simulink model "batt_test"  (Simulink 7.8)
settings: Solver=ode3  StartTime=0.0  StopTime=20  FixedStep=80e-6  RelTol=1e-3
PostLoadFcn:
  | Ts=80e-6;
InitFcn:
  | Ts=80e-6;
values from neighbouring files (symbols this model uses):
  batt_esr = (max_power*0.01)/(max_power/Vdc_nom)^2    [BES_init.m]
  C = IacRMS*18e-6    [BES_init.m]
  f = 60    [global_parameters.m]
  I_ki = 0.03    [BES_init.m]
  I_kp = 0.05    [BES_init.m]
  Iac_max = IGBT_currents(possible_currents(1))    [BES_init.m]
  Id_at_max = 3*max_pow*(2/3)/Vd_at_max    [BES_init.m]
  Iq_at_max = 3*max_pow*(2/3)/Vq_at_max    [BES_init.m]
  L = Vdc_nom/(IacRMS*0.2/(2/fs))    [BES_init.m]
  PLL_Ki = 0.001*30    (= 0.03)    [BES_init.m]
  PLL_Kp = .001*30    (= 0.03)    [BES_init.m]
  PLL_time_step = Ts    (= 8e-05)    [global_parameters.m]
  Roff = 1e7    (= 10000000)    [BES_init.m]
  Td_es_min = Ts    (= 8e-05)    [global_parameters.m]
  Tds = Ts    (= 8e-05)    [global_parameters.m]
  Vdc_max = IGBT_voltages(possible_voltages(1))    [BES_init.m]
undefined symbols (not defined in the file or in its folder): D, DiscIntNeverNeededParam
libraries: simulink x25, powerlib x20, simulink_extras x10, cstextras x9, powerlib_extras x8, modbus_lib x6, dynamic_load_lib x1, dspsigops x1
(part 2 of 2)

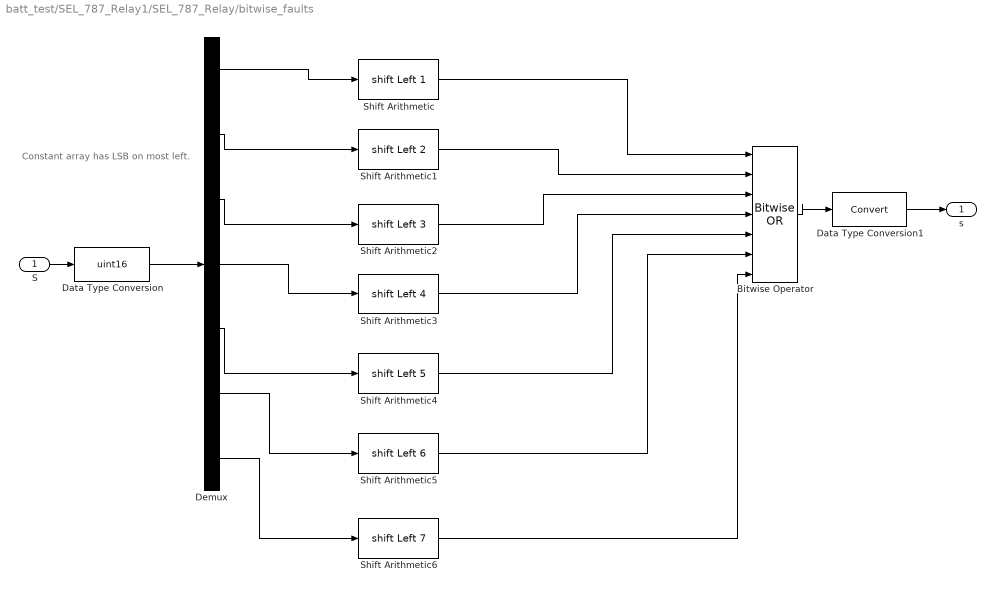
== system batt_test/SEL_787_Relay1/SEL_787_Relay/bitwise_faults ==
  note: Constant array has LSB on most left.
  S : Inport
  Bitwise Operator : simulink/Logic and Bit Operations/Bitwise Operator  logicop=OR  UseBitMask=off  NumInputPorts=7  BitMask=bin2dec('11011001')  BitMaskRealWorld=Stored Integer
  Data Type Conversion : DataTypeConversion  OutDataTypeStr=uint16
  Data Type Conversion1 : DataTypeConversion
  Demux : Demux  Outputs=7
  Shift Arithmetic : ArithShift  BitShiftNumber=1  BitShiftDirection=Left
  Shift Arithmetic1 : ArithShift  BitShiftNumber=2  BitShiftDirection=Left
  Shift Arithmetic2 : ArithShift  BitShiftNumber=3  BitShiftDirection=Left
  Shift Arithmetic3 : ArithShift  BitShiftNumber=4  BitShiftDirection=Left
  Shift Arithmetic4 : ArithShift  BitShiftNumber=5  BitShiftDirection=Left
  Shift Arithmetic5 : ArithShift  BitShiftNumber=6  BitShiftDirection=Left
  Shift Arithmetic6 : ArithShift  BitShiftNumber=7  BitShiftDirection=Left
  s : Outport
  wires:
  Demux/7 -> Shift Arithmetic6/1
  Shift Arithmetic6/1 -> Bitwise Operator/7
  Shift Arithmetic5/1 -> Bitwise Operator/6
  Shift Arithmetic4/1 -> Bitwise Operator/5
  Shift Arithmetic3/1 -> Bitwise Operator/4
  Shift Arithmetic2/1 -> Bitwise Operator/3
  Shift Arithmetic1/1 -> Bitwise Operator/2
  Shift Arithmetic/1 -> Bitwise Operator/1
  Demux/6 -> Shift Arithmetic5/1
  Demux/5 -> Shift Arithmetic4/1
  Demux/4 -> Shift Arithmetic3/1
  Demux/3 -> Shift Arithmetic2/1
  Demux/2 -> Shift Arithmetic1/1
  Demux/1 -> Shift Arithmetic/1
  Data Type Conversion1/1 -> s/1
  Bitwise Operator/1 -> Data Type Conversion1/1
  S/1 -> Data Type Conversion/1
  Data Type Conversion/1 -> Demux/1

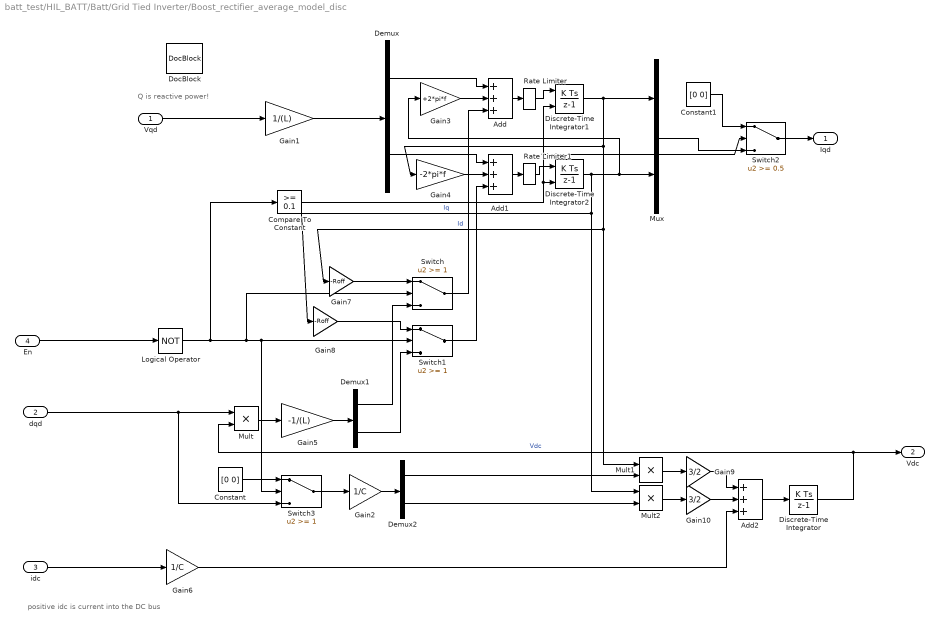
== system batt_test/HIL_BATT/Batt/Grid Tied Inverter/Boost_rectifier_average_model_disc ==
  note: positive idc is current into the DC bus
  note: Q is reactive power!
  Vqd : Inport
  dqd : Inport  Port=2  PortDimensions=2
  idc : Inport  Port=3
  En : Inport  Port=4  OutDataTypeStr=boolean
  Add : Sum  Inputs=+++
  Add1 : Sum  Inputs=+++
  Add2 : Sum  Inputs=+++
  Compare To Constant : simulink/Logic and Bit Operations/Compare To Constant  relop=>=  const=0.1  OutDataTypeStr=uint8
  Constant : Constant  Value=[0 0]
  Constant1 : Constant  Value=[0 0]
  Demux : Demux  Outputs=2
  Demux1 : Demux  Outputs=2
  Demux2 : Demux  Outputs=2
  Discrete-Time Integrator : DiscreteIntegrator  InitialCondition=Vdc_nom  InitialConditionMode=State only (most efficient)  SampleTime=Tds  ICPrevOutput=DiscIntNeverNeededParam  ICPrevScaledInput=DiscIntNeverNeededParam
  Discrete-Time Integrator1 : DiscreteIntegrator  ExternalReset=rising  InitialConditionMode=State only (most efficient)  SampleTime=Tds  ICPrevOutput=DiscIntNeverNeededParam  ICPrevScaledInput=DiscIntNeverNeededParam
  Discrete-Time Integrator2 : DiscreteIntegrator  ExternalReset=rising  InitialConditionMode=State only (most efficient)  SampleTime=Tds  ICPrevOutput=DiscIntNeverNeededParam  ICPrevScaledInput=DiscIntNeverNeededParam
  DocBlock : simulink/Model-Wide Utilities/DocBlock  DocumentType=Text
  Gain1 : Gain  Gain=1/(L)
  Gain10 : Gain  Gain=3/2
  Gain2 : Gain  Gain=1/C
  Gain3 : Gain  Gain=+2*pi*f
  Gain4 : Gain  Gain=-2*pi*f
  Gain5 : Gain  Gain=-1/(L)
  Gain6 : Gain  Gain=1/C
  Gain7 : Gain  Gain=-Roff
  Gain8 : Gain  Gain=-Roff
  Gain9 : Gain  Gain=3/2
  Logical Operator : Logic  Operator=NOT  AllPortsSameDT=off  OutDataTypeStr=boolean
  Mult : Product  Inputs=**
  Mult1 : Product  Inputs=**
  Mult2 : Product  Inputs=**
  Mux : Mux  Inputs=2
  Rate Limiter : RateLimiter  RisingSlewLimit=1e6  FallingSlewLimit=-1e6  SampleTimeMode=inherited
  Rate Limiter1 : RateLimiter  RisingSlewLimit=1e6  FallingSlewLimit=-1e6  SampleTimeMode=inherited
  Switch : Switch  Threshold=1
  Switch1 : Switch  Threshold=1
  Switch2 : Switch  Threshold=0.5
  Switch3 : Switch  Threshold=1
  Iqd : Outport
  Vdc : Outport  Port=2
  wires:
  Mux/1 -> Switch2/3
  Constant1/1 -> Switch2/1
  Switch2/1 -> Iqd/1
  Compare To Constant/1 -> Discrete-Time Integrator2/2, Switch2/2, Discrete-Time Integrator1/2
  Vqd/1 -> Gain1/1
  dqd/1 -> Switch3/3, Mult/1
  Discrete-Time Integrator/1 -> Mult/2, Vdc/1  "Vdc"
  Demux/2 -> Add1/1
  Demux2/1 -> Mult1/2
  Gain3/1 -> Add/2
  Gain4/1 -> Add1/2
  Demux1/1 -> Switch/3
  Gain2/1 -> Demux2/1
  Gain6/1 -> Add2/3
  Gain10/1 -> Add2/2
  Logical Operator/1 -> Switch3/2, Switch1/2, Switch/2, Compare To Constant/1
  Switch3/1 -> Gain2/1
  Discrete-Time Integrator1/1 -> Gain7/1, Mult1/1, Gain4/1, Mux/1  "Id"
  En/1 -> Logical Operator/1
  Demux/1 -> Add/1
  Gain7/1 -> Switch/1
  Add2/1 -> Discrete-Time Integrator/1
  Mult/1 -> Gain5/1
  idc/1 -> Gain6/1
  Demux2/2 -> Mult2/2
  Gain9/1 -> Add2/1
  Constant/1 -> Switch3/1
  Mult2/1 -> Gain10/1
  Gain5/1 -> Demux1/1
  Gain1/1 -> Demux/1
  Switch/1 -> Add/3
  Add/1 -> Rate Limiter/1
  Switch1/1 -> Add1/3
  Mult1/1 -> Gain9/1
  Demux1/2 -> Switch1/3
  Discrete-Time Integrator2/1 -> Gain8/1, Mult2/1, Gain3/1, Mux/2  "Iq"
  Gain8/1 -> Switch1/1
  Add1/1 -> Rate Limiter1/1
  Rate Limiter/1 -> Discrete-Time Integrator1/1
  Rate Limiter1/1 -> Discrete-Time Integrator2/1

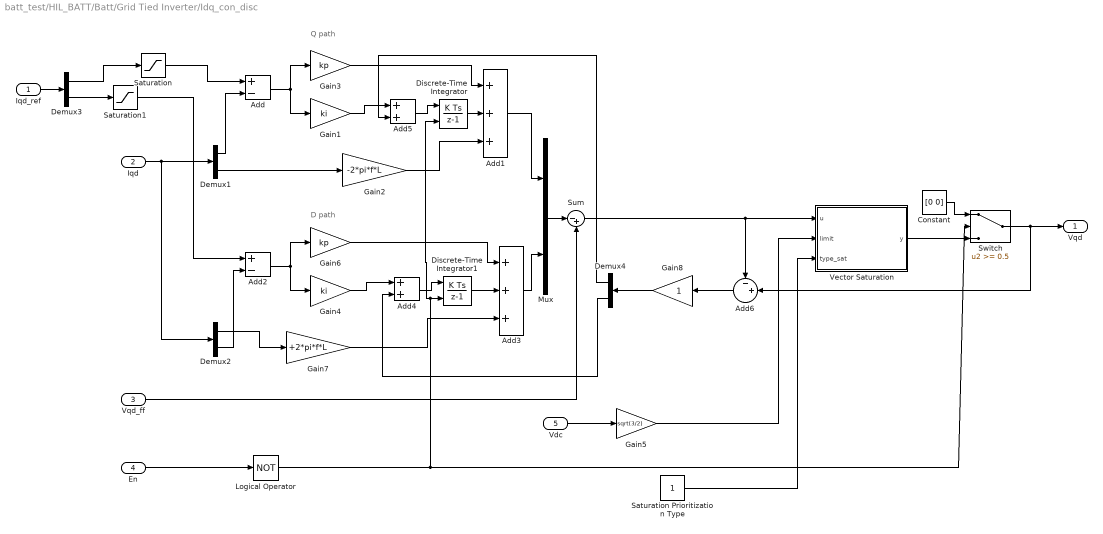
== system batt_test/HIL_BATT/Batt/Grid Tied Inverter/Idq_con_disc ==
  note: D path
  note: Q path
  Iqd_ref : Inport
  Iqd : Inport  Port=2
  Vqd_ff : Inport  Port=3  PortDimensions=2
  En : Inport  Port=4  OutDataTypeStr=boolean  PortDimensions=1
  Vdc : Inport  Port=5  PortDimensions=1
  Add : Sum  Inputs=+-
  Add1 : Sum  Inputs=+++
  Add2 : Sum  Inputs=+-
  Add3 : Sum  Inputs=+++
  Add4 : Sum
  Add5 : Sum
  Add6 : Sum  Inputs=-+|
  Constant : Constant  Value=[0 0]
  Demux{1..4} (4 alike) : Demux  Outputs=2
  Discrete-Time Integrator : DiscreteIntegrator  ExternalReset=level  InitialConditionMode=State only (most efficient)  SampleTime=Td_es_min  ICPrevOutput=DiscIntNeverNeededParam  ICPrevScaledInput=DiscIntNeverNeededParam
  Discrete-Time Integrator1 : DiscreteIntegrator  ExternalReset=level  InitialConditionMode=State only (most efficient)  SampleTime=Td_es_min  ICPrevOutput=DiscIntNeverNeededParam  ICPrevScaledInput=DiscIntNeverNeededParam
  Gain1 : Gain  Gain=ki
  Gain2 : Gain  Gain=-2*pi*f*L
  Gain3 : Gain  Gain=kp
  Gain4 : Gain  Gain=ki
  Gain5 : Gain  Gain=sqrt(3/2)
  Gain6 : Gain  Gain=kp
  Gain7 : Gain  Gain=+2*pi*f*L
  Gain8 : Gain
  Logical Operator : Logic  Operator=NOT  AllPortsSameDT=off  OutDataTypeStr=boolean
  Mux : Mux  Inputs=2
  Saturation : Saturate  UpperLimit=iq_max  LowerLimit=-iq_max
  Saturation Prioritization Type : Constant
  Saturation1 : Saturate  UpperLimit=id_max  LowerLimit=-id_max
  Sum : Sum  Inputs=|-+
  Switch : Switch  Threshold=0.5
  Vector Saturation : MATLAB Function  TreatAsAtomicUnit=on
  Vqd : Outport
  wires:
  Constant/1 -> Switch/1
  Vector Saturation/1(y) -> Switch/3
  Logical Operator/1 -> Switch/2, Discrete-Time Integrator1/2, Discrete-Time Integrator/2
  Switch/1 -> Add6/2, Vqd/1
  Vdc/1 -> Gain5/1
  Add6/1 -> Gain8/1
  Gain5/1 -> Vector Saturation/2(limit)
  Saturation Prioritization Type/1 -> Vector Saturation/3(type_sat)
  Vqd_ff/1 -> Sum/2
  Demux2/1 -> Gain7/1
  Demux4/1 -> Add5/2
  Saturation/1 -> Add/1
  Saturation1/1 -> Add2/1
  Iqd_ref/1 -> Demux3/1
  Gain8/1 -> Demux4/1
  Add2/1 -> Gain6/1, Gain4/1
  Demux1/2 -> Gain2/1
  Demux1/1 -> Add/2
  Gain3/1 -> Add1/1
  Sum/1 -> Add6/1, Vector Saturation/1(u)
  Add1/1 -> Mux/1
  Gain4/1 -> Add4/1
  Add5/1 -> Discrete-Time Integrator/1
  Demux3/1 -> Saturation/1
  Add4/1 -> Discrete-Time Integrator1/1
  Iqd/1 -> Demux1/1, Demux2/1
  Discrete-Time Integrator/1 -> Add1/2
  Demux3/2 -> Saturation1/1
  Gain2/1 -> Add1/3
  Gain1/1 -> Add5/1
  En/1 -> Logical Operator/1
  Add3/1 -> Mux/2
  Demux2/2 -> Add2/2
  Gain7/1 -> Add3/3
  Discrete-Time Integrator1/1 -> Add3/2
  Mux/1 -> Sum/1
  Demux4/2 -> Add4/2
  Gain6/1 -> Add3/1
  Add/1 -> Gain3/1, Gain1/1

== system batt_test/HIL_BATT/Batt/Grid Tied Inverter/Latch ==
  In1 : Inport
  Reset : Inport  Port=2
  Demux : Demux  Outputs=6
  Logical Operator6 : Logic  Operator=NOT  AllPortsSameDT=off  OutDataTypeStr=boolean
  Mux : Mux  Inputs=6
  S-R Flip-Flop{,1..5} (6 alike) : simulink_extras/Flip Flops/S-R Flip-Flop  initial_condition=0
  Out1 : Outport
  wires:
  S-R Flip-Flop5/1 -> Mux/6  "Vac"
  S-R Flip-Flop4/1 -> Mux/5  "PLL"
  S-R Flip-Flop3/1 -> Mux/4  "Vdc"
  Demux/6 -> S-R Flip-Flop5/1
  Demux/5 -> S-R Flip-Flop4/1
  Demux/4 -> S-R Flip-Flop3/1
  Demux/3 -> S-R Flip-Flop2/1
  S-R Flip-Flop2/1 -> Mux/3  "Ic"
  S-R Flip-Flop/1 -> Mux/1  "Ia"
  Mux/1 -> Out1/1  "Faults"
  Demux/1 -> S-R Flip-Flop/1
  In1/1 -> Demux/1
  S-R Flip-Flop1/1 -> Mux/2  "Ib"
  Demux/2 -> S-R Flip-Flop1/1
  Reset/1 -> Logical Operator6/1
  Logical Operator6/1 -> S-R Flip-Flop5/2, S-R Flip-Flop4/2, S-R Flip-Flop3/2, S-R Flip-Flop2/2, S-R Flip-Flop/2, S-R Flip-Flop1/2

== system batt_test/HIL_BATT/Batt/Grid Tied Inverter/Modulator ==
  Vqd : Inport
  Vdc : Inport  Port=2
  Delay : Delay  DelayLength=1  InitialCondition=[0 0]  SampleTime=Td_es_min
  IC : InitialCondition  Value=Vdc_nom
  Mult1 : Product  Inputs=*/
  Saturation : Saturate  UpperLimit=1  LowerLimit=-1
  dqd : Outport
  wires:
  Mult1/1 -> Saturation/1
  Saturation/1 -> Delay/1
  Vqd/1 -> Mult1/1
  Vdc/1 -> IC/1
  IC/1 -> Mult1/2
  Delay/1 -> dqd/1

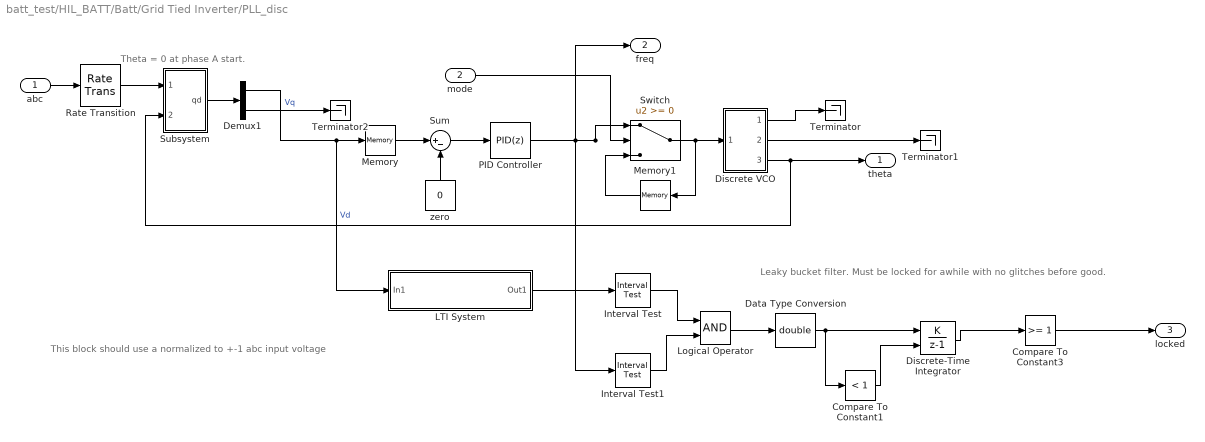
== system batt_test/HIL_BATT/Batt/Grid Tied Inverter/PLL_disc ==
  note: Leaky bucket filter. Must be locked for awhile with no glitches before good.
  note: Theta = 0 at phase A start.
  note: This block should use a normalized to +-1 abc input voltage
  abc : Inport  PortDimensions=3
  mode : Inport  Port=2
  Compare To Constant1 : simulink/Logic and Bit Operations/Compare To Constant  relop=<  const=1  OutDataTypeStr=boolean
  Compare To Constant3 : simulink/Logic and Bit Operations/Compare To Constant  relop=>=  const=1  OutDataTypeStr=boolean
  Data Type Conversion : DataTypeConversion  OutDataTypeStr=double
  Demux1 : Demux  Outputs=2
  Discrete VCO : Subsystem
  Discrete-Time Integrator : DiscreteIntegrator  IntegratorMethod=Accumulation: Forward Euler  gainval=Td_es_min/0.5  ExternalReset=rising  SampleTime=Td_es_min  LimitOutput=on  UpperSaturationLimit=1  LowerSaturationLimit=0  ICPrevOutput=DiscIntNeverNeededParam  ICPrevScaledInput=DiscIntNeverNeededParam
  Interval Test : simulink/Logic and Bit Operations/Interval Test  IntervalClosedRight=on  uplimit=PLL_lock_window  IntervalClosedLeft=on  lowlimit=-PLL_lock_window  OutDataTypeStr=boolean
  Interval Test1 : simulink/Logic and Bit Operations/Interval Test  IntervalClosedRight=on  uplimit=2*pi*f*(1+PLL_freq_range)  IntervalClosedLeft=on  lowlimit=2*pi*f*(1-PLL_freq_range)  OutDataTypeStr=boolean
  LTI System : Subsystem  BlockChoice=CSS  mask(LTI Block){sys=c2d(tf(1,[1/(f*2*2*pi),1]),Td_es_min), IC=[]}
      mask prompts: sys "LTI system variable"; IC "Initial states (state-space only)"
      mask help:
      | The LTI System block accepts both continuous and discrete LTI models as defined in the Control System Toolbox. Transfer function, state-space, and zero-pole-gain formats are all supported in this block.
      |
      | Note: Initial states are only meaningful for state-space systems.
      mask init: same as batt_test/Low-pass
      mask Help:
      | The LTI System block accepts any of the three standard LTI models described in the Control System Toolbox: transfer function, zero/pole/gain, or state space. Internally, LTI models will be converted to their state space equivalent for evaluation.
      | <p>
      | In the editable text box labeled <b>LTI System Variable</b>, enter a valid LTI model.
      | <p>
      | In the editable text box labeled <b>Initial States</b> enter the initial state vector.  Initial states are only valid for state-space systems.
      | <p>
      | See also TF, ZPK, SS, LTIMODELS.
      mask CallbackString: ltimask('MaskLTICallback',gcb);|
      mask Display: disp(sysname)
  Logical Operator : Logic  AllPortsSameDT=off  OutDataTypeStr=boolean
  Memory : Memory
  Memory1 : Memory
  PID Controller : simulink/Continuous/PID Controller  Controller=PID  TimeDomain=Discrete-time  SampleTime=PLL_time_step  IntegratorMethod=Forward Euler  FilterMethod=Forward Euler  Form=Parallel  P=PLL_Kp  I=PLL_Ki  D=0  N=100  InitialConditionSource=internal  InitialConditionForIntegrator=2*pi*f  InitialConditionForFilter=0  ExternalReset=none  ZeroCross=off  LimitOutput=on  UpperSaturationLimit=2*pi*(f*(1+PLL_freq_range))  LowerSaturationLimit=2*pi*(f*(1-PLL_freq_range))  LinearizeAsGain=on  AntiWindupMode=clamping  Kb=1  TrackingMode=off  Kt=1  PParamMin=[]  PParamMax=[]  IParamMin=[]  IParamMax=[]  DParamMin=[]  DParamMax=[]  NParamMin=[]  NParamMax=[]  KbParamMin=[]  KbParamMax=[]  KtParamMin=[]  KtParamMax=[]  POutMin=[]  POutMax=[]  IOutMin=[]  IOutMax=[]  DOutMin=[]  DOutMax=[]  NOutMin=[]  NOutMax=[]  KbOutMin=[]  KbOutMax=[]  KtOutMin=[]  KtOutMax=[]  IntegratorOutMin=[]  IntegratorOutMax=[]  FilterOutMin=[]  FilterOutMax=[]  SumOutMin=[]  SumOutMax=[]  SumI1OutMin=[]  SumI1OutMax=[]  SumI2OutMin=[]  SumI2OutMax=[]  SumI3OutMin=[]  SumI3OutMax=[]  SumDOutMin=[]  SumDOutMax=[]  SaturationOutMin=[]  SaturationOutMax=[]  IntegratorContinuousStateAttributes=''  IntegratorStateMustResolveToSignalObject=off  IntegratorRTWStateStorageClass=Auto  FilterContinuousStateAttributes=''  FilterStateMustResolveToSignalObject=off  FilterRTWStateStorageClass=Auto
  Rate Transition : RateTransition  OutPortSampleTime=PLL_time_step
  Subsystem : Subsystem
  Sum : Sum  Inputs=|+-
  Switch : Switch
  Terminator : Terminator
  Terminator1 : Terminator
  Terminator2 : Terminator
  zero : Constant  Value=0
  theta : Outport
  freq : Outport  Port=2
  locked : Outport  Port=3
  wires:
  Memory/1 -> Sum/1
  Compare To Constant3/1 -> locked/1
  Compare To Constant1/1 -> Discrete-Time Integrator/2
  Data Type Conversion/1 -> Discrete-Time Integrator/1, Compare To Constant1/1
  Discrete-Time Integrator/1 -> Compare To Constant3/1
  Demux1/2 -> Terminator2/1  "Vq"
  Demux1/1 -> Memory/1, LTI System/1(In1)  "Vd"
  Discrete VCO/3(theta) -> theta/1, Subsystem/2(theta)
  Logical Operator/1 -> Data Type Conversion/1
  Rate Transition/1 -> Subsystem/1(abc)
  zero/1 -> Sum/2
  Interval Test/1 -> Logical Operator/1
  Interval Test1/1 -> Logical Operator/2
  abc/1 -> Rate Transition/1
  Subsystem/1(qd) -> Demux1/1
  Discrete VCO/1(Cos) -> Terminator/1
  PID Controller/1 -> Interval Test1/1, freq/1, Switch/1
  Discrete VCO/2(Sin) -> Terminator1/1
  LTI System/1(Out1) -> Interval Test/1
  Sum/1 -> PID Controller/1
  Switch/1 -> Memory1/1, Discrete VCO/1(In1)
  Memory1/1 -> Switch/3
  mode/1 -> Switch/2

== system batt_test/HIL_BATT/Batt/Grid Tied Inverter/RMS_Calculator ==
  Signal : Inport
  Discrete  Mean value6 : powerlib_extras/Discrete Measurements/Discrete  Mean value  Freq=60/4  Vinit=0  Ts=Ts
  Memory : Memory
  Product3 : Product  RndMeth=Zero
  Signed Sqrt : Sqrt  SaturateOnIntegerOverflow=on
  RMS_Signal : Outport
  wires:
  Memory/1 -> Discrete  Mean value6/1
  Signed Sqrt/1 -> RMS_Signal/1
  Discrete  Mean value6/1 -> Signed Sqrt/1
  Product3/1 -> Memory/1
  Signal/1 -> Product3/2, Product3/1

== system batt_test/HIL_BATT/Batt/Grid Tied Inverter/Subsystem ==
  qd : Inport  OutDataTypeStr=double  PortDimensions=2
  theta : Inport  Port=2  OutDataTypeStr=double  PortDimensions=1
  Mux : Mux  Inputs=3
  Mux1 : Mux  Inputs=2
  qd>a : Fcn  Expr=u[1]*cos(u[3])-u[2]*sin(u[3])
  qd>b : Fcn  Expr=u[1]*cos(u[3]-2*pi/3)-u[2]*sin(u[3]-2*pi/3)
  qd>c : Fcn  Expr=u[1]*cos(u[3]+2*pi/3)-u[2]*sin(u[3]+2*pi/3)
  abc : Outport  OutDataTypeStr=double  PortDimensions=3
  wires:
  qd>a/1 -> Mux/1
  Mux1/1 -> qd>a/1, qd>b/1, qd>c/1
  theta/1 -> Mux1/2
  qd>c/1 -> Mux/3
  qd/1 -> Mux1/1
  qd>b/1 -> Mux/2
  Mux/1 -> abc/1

== system batt_test/HIL_BATT/Batt/Grid Tied Inverter/Subsystem1 ==
  abc : Inport  OutDataTypeStr=double  PortDimensions=3
  theta : Inport  Port=2  OutDataTypeStr=double  PortDimensions=1
  Mux : Mux  Inputs=2
  Mux1 : Mux  Inputs=2
  abc>d : Fcn  Expr=2/3*(u[1]*cos(u[4])+u[2]*cos(u[4]-2*pi/3)+u[3]*cos(u[4]+2*pi/3))
  abc>q : Fcn  Expr=2/3*(-u[1]*sin(u[4])-u[2]*sin(u[4]-2*pi/3)-u[3]*sin(u[4]+2*pi/3))
  qd : Outport  OutDataTypeStr=double  PortDimensions=2
  wires:
  abc/1 -> Mux1/1
  theta/1 -> Mux1/2
  abc>q/1 -> Mux/2
  abc>d/1 -> Mux/1
  Mux/1 -> qd/1
  Mux1/1 -> abc>d/1, abc>q/1

== system batt_test/HIL_BATT/Batt/Grid Tied Inverter/Windowed Limit ==
  Signal : Inport
  Threshold : Inport  Port=2
  Abs : Abs
  Relational Operator2 : RelationalOperator  Operator=>  OutDataTypeStr=boolean
  TestOut : Outport
  wires:
  Signal/1 -> Abs/1
  Threshold/1 -> Relational Operator2/2
  Relational Operator2/1 -> TestOut/1
  Abs/1 -> Relational Operator2/1

== system batt_test/SEL_787_Relay1/SEL_787_Relay/Relay 25 - Sync Check - RS/Freq_Comparator ==
  f_grid : Inport
  f_gen : Inport  Port=2
  Abs : Abs
  Compare To Constant2 : simulink/Logic and Bit Operations/Compare To Constant  relop=<=  const=0.5  OutDataTypeStr=uint8
  Fcn2 : Fcn  Expr=u(2)-u(1)
  Mux1 : Mux  Inputs=2
  Locked : Outport
  wires:
  Compare To Constant2/1 -> Locked/1
  f_grid/1 -> Mux1/1
  f_gen/1 -> Mux1/2
  Fcn2/1 -> Abs/1
  Mux1/1 -> Fcn2/1
  Abs/1 -> Compare To Constant2/1

== system batt_test/SEL_787_Relay1/SEL_787_Relay/Relay 25 - Sync Check - RS/Phase_Comparator ==
  wt_grid : Inport
  wt_gen : Inport  Port=2
  Compare To Constant1 : simulink/Logic and Bit Operations/Compare To Constant  relop=<=  const=12  OutDataTypeStr=uint8
  Constant3 : Constant  Value=2*pi
  Fcn3 : Fcn  Expr=abs(u(2)-u(1))  SampleTime=Ts
  Math Function : Math  Operator=mod  SampleTime=Ts  SaturateOnIntegerOverflow=on
  Mux3 : Mux  Inputs=2
  Radians to Degrees : simulink_extras/Transformations/Radians to Degrees
  Unwrap : dspsigops/Unwrap  tol=pi  InputProcessing=Columns as channels (frame based)  running=off
  Locked : Outport
  wires:
  Unwrap/1 -> Fcn3/1
  Math Function/1 -> Unwrap/1
  Compare To Constant1/1 -> Locked/1  "bool"
  wt_gen/1 -> Mux3/2
  wt_grid/1 -> Mux3/1
  Fcn3/1 -> Radians to Degrees/1  "diff"
  Mux3/1 -> Math Function/1
  Constant3/1 -> Math Function/2
  Radians to Degrees/1 -> Compare To Constant1/1  "R2D"

== system batt_test/SEL_787_Relay1/SEL_787_Relay/Relay 25 - Sync Check - RS/RMS ==
  s : Inport
  Discrete  Mean value6 : powerlib_extras/Discrete Measurements/Discrete  Mean value  Freq=60  Vinit=0  Ts=Ts
  Product3 : Product  RndMeth=Zero
  Signed Sqrt : Sqrt  SaturateOnIntegerOverflow=on
  S : Outport
  wires:
  Signed Sqrt/1 -> S/1
  Discrete  Mean value6/1 -> Signed Sqrt/1
  Product3/1 -> Discrete  Mean value6/1
  s/1 -> Product3/2, Product3/1

== system batt_test/SEL_787_Relay1/SEL_787_Relay/Relay 25 - Sync Check - RS/Voltage_Comparator ==
  V_bus : Inport
  V_line : Inport  Port=2
  3% of the nominal VRMSLL : simulink/Logic and Bit Operations/Compare To Constant  relop=<=  const=VRMSLL*0.03  OutDataTypeStr=uint8
  Discrete Transfer Fcn : DiscreteTransferFcn  Numerator=[0.0004999]  Denominator=[1 -0.9995]  SampleTime=-1
  Fcn2 : Fcn  Expr=abs(u(2)-u(1))
  Mux1 : Mux  Inputs=2
  Locked : Outport
  wires:
  V_bus/1 -> Mux1/1
  V_line/1 -> Mux1/2
  Discrete Transfer Fcn/1 -> 3% of the nominal VRMSLL/1  "flt"
  3% of the nominal VRMSLL/1 -> Locked/1  "thshld"
  Fcn2/1 -> Discrete Transfer Fcn/1  "diff"
  Mux1/1 -> Fcn2/1

== system batt_test/SEL_787_Relay1/SEL_787_Relay/Relay 25 - Sync Check - RS/set of 1ph PLLs ==
  V_bus : Inport
  V_line : Inport  Port=2
  Discrete 1-phase PLL : powerlib_extras/Discrete  Control Blocks/Discrete 1-phase PLL  Fmin=45  Par_Init=[0 60]  ParK=[ 180 3200 1]  Ts=Ts  AGC=on
  Discrete 1-phase PLL1 : powerlib_extras/Discrete  Control Blocks/Discrete 1-phase PLL  Fmin=45  Par_Init=[0 60]  ParK=[ 180 3200 1]  Ts=Ts  AGC=on
  Gain : Gain  Gain=1/VRMSLL
  Gain1 : Gain  Gain=1/VRMSLL
  Terminator : Terminator
  Terminator1 : Terminator
  f_bus : Outport
  f_line : Outport  Port=2
  wt_bus : Outport  Port=3
  wt_line : Outport  Port=4
  wires:
  Gain1/1 -> Discrete 1-phase PLL1/1
  V_bus/1 -> Gain1/1
  Gain/1 -> Discrete 1-phase PLL/1
  V_line/1 -> Gain/1
  Discrete 1-phase PLL1/1 -> f_bus/1
  Discrete 1-phase PLL1/2 -> wt_bus/1
  Discrete 1-phase PLL/1 -> f_line/1
  Discrete 1-phase PLL/2 -> wt_line/1
  Discrete 1-phase PLL/3 -> Terminator/1
  Discrete 1-phase PLL1/3 -> Terminator1/1

== system batt_test/HIL_BATT/Batt/Grid Tied Inverter/PLL_disc/Discrete VCO ==
  note: VCO
  In1 : Inport
  Constant : Constant  Value=2*pi
  Discrete-Time Integrator : DiscreteIntegrator  InitialConditionMode=State only (most efficient)  SampleTime=Td_es_min  ICPrevOutput=DiscIntNeverNeededParam  ICPrevScaledInput=DiscIntNeverNeededParam
  Gain1 : Gain  OutDataTypeStr=double
  Math Function : Math  Operator=mod  SaturateOnIntegerOverflow=on
  Scope2 : Scope
      settings: TimeRange=0.1  YMin=0  YMax=70000
  cos1 : Trigonometry  Operator=cos
  sin1 : Trigonometry
  Cos : Outport
  Sin : Outport  Port=2
  theta : Outport  Port=3
  wires:
  Math Function/1 -> sin1/1, cos1/1, theta/1, Scope2/1
  Discrete-Time Integrator/1 -> Math Function/1
  Gain1/1 -> Discrete-Time Integrator/1
  Constant/1 -> Math Function/2
  sin1/1 -> Sin/1
  cos1/1 -> Cos/1
  In1/1 -> Gain1/1

== system batt_test/HIL_BATT/Batt/Grid Tied Inverter/PLL_disc/LTI System ==
  In1 : Inport
  IO Delay : cstextras/Integer Delay (masked)  Td=Tdio  u0=0  Ts=Ts
  Input Delay : cstextras/Integer Delay (masked)  Td=Tdi  u0=0  Ts=Ts
  Internal : DiscreteStateSpace  A=D.a  B=D.b  C=D.c  D=D.d  SampleTime=Ts
  Output Delay : cstextras/Integer Delay (masked)  Td=Tdo  u0=0  Ts=Ts
  Out1 : Outport  InitialOutput=0
  wires:
  In1/1 -> Input Delay/1
  Output Delay/1 -> Out1/1
  Input Delay/1 -> Internal/1
  Internal/1 -> IO Delay/1
  IO Delay/1 -> Output Delay/1

== system batt_test/HIL_BATT/Batt/Grid Tied Inverter/PLL_disc/Subsystem ==
  abc : Inport  OutDataTypeStr=double  PortDimensions=3
  theta : Inport  Port=2  OutDataTypeStr=double  PortDimensions=1
  Mux : Mux  Inputs=2
  Mux1 : Mux  Inputs=2
  abc>d : Fcn  Expr=2/3*(u[1]*cos(u[4])+u[2]*cos(u[4]-2*pi/3)+u[3]*cos(u[4]+2*pi/3))
  abc>q : Fcn  Expr=2/3*(-u[1]*sin(u[4])-u[2]*sin(u[4]-2*pi/3)-u[3]*sin(u[4]+2*pi/3))
  qd : Outport  OutDataTypeStr=double  PortDimensions=2
  wires:
  Mux1/1 -> abc>q/1, abc>d/1
  Mux/1 -> qd/1
  abc>d/1 -> Mux/1
  abc>q/1 -> Mux/2
  theta/1 -> Mux1/2
  abc/1 -> Mux1/1

== matlab function HIL_BATT/Batt/Grid Tied Inverter/Idq_con_disc/Vector Saturation ==
  data: u input double; y output double; limit input double; type_sat input double
function y = fcn(u, limit, type_sat)
% When the magnitude is of u is greater than limit prioritize the
% saturation to u(type_sat) dimension.  u is two dimensional input.
%#codegen
y=zeros(2,1); % required initialization
u_sign=sign(u);

if(abs(u(1)) > limit)
    u(1) = u_sign(1).*limit;
end
if(abs(u(2)) > limit)
    u(2) =  u_sign(2).*limit;
end
if(u(1)^2 + u(2)^2 > limit^2)
    if(type_sat == 1) % priority given to u(1)
        y(1) = u(1);
        y(2) = u_sign(2) .* sqrt(limit^2 - u(1)^2); 
    else  % priority given to u(2)
        y(2) = u(2);
        y(1) =  u_sign(1) .* sqrt(limit^2 - u(2)^2); 
    end
else
    y = u;
end

== matlab function SEL_787_Relay1/SEL_787_Relay/trip_out mng ==
  data: Ts input double; bool_R25 input double; op_mode_in input double; trip_out output double; trip_in input double; synch_check_time input double
function trip_out = opModeChk(Ts, bool_R25, op_mode_in, trip_in, synch_check_time)
%#codegen

persistent n25 prev_mode prev_trip_in
if isempty(prev_mode)
    n25 = 0; % time counter
    prev_mode = 0; % initially operating on logic
    prev_trip_in = 1; % initially close
end

trip_out = trip_in * bool_R25;

% the R25 logic will be active if the breaker has been opened, and a
% forced-to-close command is applied
if (prev_mode==2 || prev_trip_in==0) && (op_mode_in==1 || op_mode_in==0) && trip_in==1
    
    % time accumulation
    n25 = n25 * bool_R25;
    n25 = n25 + bool_R25 * Ts;
    if n25 > synch_check_time
        trip_out = 1;
        % reset history values
        prev_mode = op_mode_in;
        prev_trip_in = trip_in;
    else
        prev_mode = 2;
        prev_trip_in = 0;
        trip_out = 0;
    end
    
elseif op_mode_in==2
    prev_mode = 2;
    prev_trip_in = 0;
    trip_out = 0;
    n25 = 0;
else
    n25 = 0;
end

== matlab function SEL_787_Relay1/SEL_787_Relay/Relay 25 - Sync Check - RS/deadbus fcn ==
  data: Vbus input double; y output double; Vline input double; VRMSLL input double
function y = fcn(Vbus, Vline, VRMSLL)
%#codegen
if isnan(Vbus)
    Vbus=0;
elseif isnan(Vline)
    Vline = 0;
end
threshold = 20; % voltage threshold for deadbus
% bounding open-circuit voltage at 120%
a = (Vbus>(VRMSLL*0.90)) && (Vbus<(VRMSLL*1.20)) && (Vline < threshold);
b = (Vline>(VRMSLL*0.90)) && (Vline<(VRMSLL*1.20)) && (Vbus < threshold);
y = a||b;
